simulink model "Key_life_unchanged_abnormal_check"  (R2021a)
settings: configuration reference "ART_1G_IDS_Speedgoat" (kept outside this file)
libraries: simulink x1
settings Model: DataDictionary=Key_Life_Unchanged_Abnormal_Check.sldd  Creator=xinrui  LastModifiedBy=xinrui
settings ConfigSetRef: SourceName=ART_1G_IDS_Speedgoat

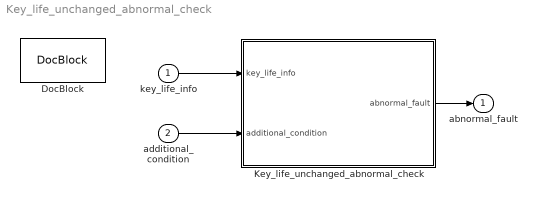
== system Key_life_unchanged_abnormal_check ==
  key_life_info : Inport  OutDataTypeStr=Bus: Key_Life_Info  PortDimensions=1
  additional_condition : Inport  Port=2  OutDataTypeStr=Enum: Validation  PortDimensions=1
  DocBlock : simulink/Model-Wide Utilities/DocBlock  DocumentType=HTML  mask(DocBlock){}
      mask Display:
      | plot([.8 0 0 1 1 .8 .8 1],[1 1 0 0 .8 1 .8 .8]);
      | text(.5,.6,'CHANGELOG','horizontalalignment','center');
      | text(.95,.05,get_param(gcb,'DocumentType'),'verticalalignment','bottom','horizontalalignment','right');
  Key_life_unchanged_abnormal_check : Stateflow chart  TreatAsAtomicUnit=on
  abnormal_fault : Outport  OutDataTypeStr=Enum: Validation  PortDimensions=1
  wires:
  Key_life_unchanged_abnormal_check/1(abnormal_fault) -> abnormal_fault/1
  key_life_info/1 -> Key_life_unchanged_abnormal_check/1(key_life_info)
  additional_condition/1 -> Key_life_unchanged_abnormal_check/2(additional_condition)

== stateflow chart Key_life_unchanged_abnormal_check/Key_life_unchanged_abnormal_check ==
  settings: updateMethod=DISCRETE
  state key_life_unchanged_abnormal_check %关键生命信号不变检测
    abnormal_condition = EPSILON > fabs(double(key_life_info.value_current) - double(key_life_info.value_previous));
    is_normal = Validation.Invalid == abnormal_condition || Validation.Invalid == additional_condition;
    need_observing = Validation.Valid == abnormal_condition && Validation.Valid == additional_condition;
    is_abnormal = key_life_info.unchanged_abnormal_check_times <= abnormal_check_counter;
    state normal %正常
      abnormal_fault = Validation.Invalid;
    state abnormal %异常
      abnormal_fault = Validation.Valid;
    state observation %观测
      abnormal_check_counter++;
    abnormal %异常 -> normal %正常 : [is_normal]
    (default) -> normal %正常
    observation %观测 -> normal %正常 [order 2] : [is_normal]
    normal %正常 -> observation %观测 : [need_observing]{abnormal_check_counter = 0}
    observation %观测 -> abnormal %异常 [order 1] : [is_abnormal]
  (default) -> key_life_unchanged_abnormal_check %关键生命信号不变检测 : {abnormal_check_counter = 0;}
  data: abnormal_condition local Enum: Validation; abnormal_check_counter local uint32; key_life_info input Bus: Key_Life_Info; additional_condition input Enum: Validation; abnormal_fault output Enum: Validation; EPSILON parameter double; is_abnormal local boolean; need_observing local boolean; is_normal local boolean
